simulink model "failure_detector"  (R2024b)
settings: Solver=VariableStepAuto  StartTime=0.0  StopTime=1  RelTol=1e-3
libraries: simulink x7, pil_lib x1
settings Model: Creator=bew  LastModifiedBy=bew

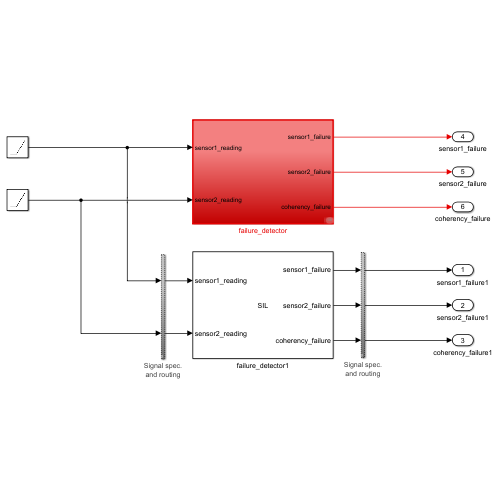
[thumbnail: Simulink's stored preview of the top-level diagram]
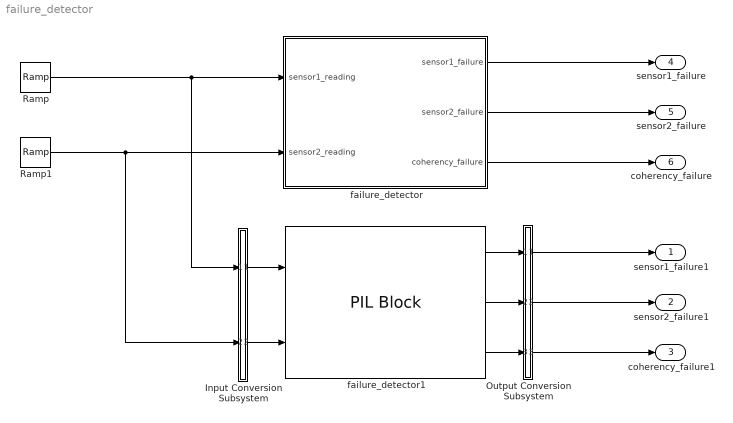
== system failure_detector ==
  Input Conversion Subsystem : Subsystem  Tag=__SLT_ICS__  Description=|
      | Signal spec.
      | and routing
      settings: AttributesFormatString=%<Description>
  Output Conversion Subsystem : Subsystem  Tag=__SLT_OCS__  Description=|
      | Signal spec.
      | and routing
      settings: AttributesFormatString=%<Description>
  Ramp : simulink/Sources/Ramp  slope=4  start=0  InitialOutput=0.5
  Ramp1 : simulink/Sources/Ramp  slope=-4  start=0  InitialOutput=4.5
  failure_detector : Subsystem  TreatAsAtomicUnit=on
  failure_detector1 : pil_lib/PIL Block  Tag=__SL_testing_harness_stub_  SimulationMode=SIL  IsTopModelPIL=off  CodeDir=D:\MBD_challenge\failure_detector_ert_rtw  AnchorDir=D:\MBD_challenge\xrel  ConfigName=Software-in-the-Loop (SIL)  XRelSourceFile=D:\MBD_challenge\failure_detector_ert_rtw\ert_main.c  XrelIsTopModelCode=on  XrelIsReusable=off  XrelDWorkNames={}  XrelDWorkTypes={}  XrelModelArgVals={}  XrelOrderedParamNames={}  XILSFunction=failure_detector_R2024b_sil  XRelNonFiniteStyle=NONFINITE_UNUSED
  sensor1_failure1 : Outport
  sensor2_failure1 : Outport  Port=2
  coherency_failure1 : Outport  Port=3
  sensor1_failure : Outport  Port=4
  sensor2_failure : Outport  Port=5
  coherency_failure : Outport  Port=6
  wires:
  Input Conversion Subsystem/1(Outport_1) -> failure_detector1/1
  Input Conversion Subsystem/2(Outport_2) -> failure_detector1/2
  failure_detector1/3 -> Output Conversion Subsystem/3(Inport_3)
  Output Conversion Subsystem/2(Outport_2) -> sensor2_failure1/1
  failure_detector1/2 -> Output Conversion Subsystem/2(Inport_2)
  Output Conversion Subsystem/1(Outport_1) -> sensor1_failure1/1
  failure_detector1/1 -> Output Conversion Subsystem/1(Inport_1)
  Output Conversion Subsystem/3(Outport_3) -> coherency_failure1/1
  failure_detector/1(sensor1_failure) -> sensor1_failure/1
  failure_detector/2(sensor2_failure) -> sensor2_failure/1
  failure_detector/3(coherency_failure) -> coherency_failure/1
  Ramp/1 -> Input Conversion Subsystem/1(Inport_1), failure_detector/1(sensor1_reading)
  Ramp1/1 -> Input Conversion Subsystem/2(Inport_2), failure_detector/2(sensor2_reading)

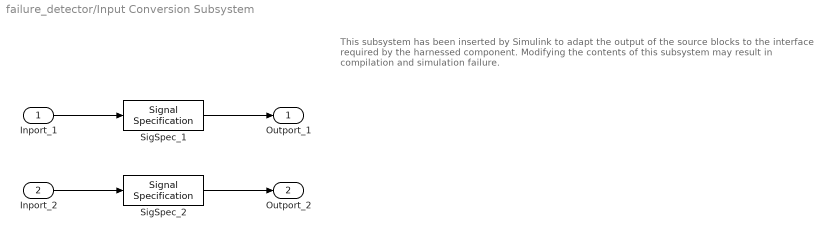
== system failure_detector/Input Conversion Subsystem ==
  note: This subsystem has been inserted by Simulink to adapt the output of the source blocks to the interface required by the harnessed component.
      |  Modifying the contents of this subsystem may result in compilation and simulation failure.
  Inport_1 : Inport
  Inport_2 : Inport  Port=2
  SigSpec_1 : SignalSpecification  OutDataTypeStr=double  Dimensions=[1]  SampleTime=0.2
  SigSpec_2 : SignalSpecification  OutDataTypeStr=double  Dimensions=[1]  SampleTime=0.2
  Outport_1 : Outport
  Outport_2 : Outport  Port=2
  wires:
  SigSpec_1/1 -> Outport_1/1
  Inport_1/1 -> SigSpec_1/1
  SigSpec_2/1 -> Outport_2/1
  Inport_2/1 -> SigSpec_2/1

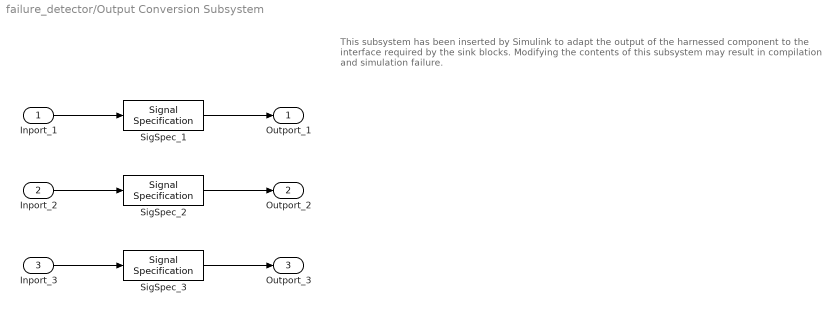
== system failure_detector/Output Conversion Subsystem ==
  note: This subsystem has been inserted by Simulink to adapt the output of the harnessed component to the interface required by the sink blocks.
      |  Modifying the contents of this subsystem may result in compilation and simulation failure.
  Inport_1 : Inport
  Inport_2 : Inport  Port=2
  Inport_3 : Inport  Port=3
  SigSpec_1 : SignalSpecification  OutDataTypeStr=boolean  Dimensions=[1]  SampleTime=0.2
  SigSpec_2 : SignalSpecification  OutDataTypeStr=boolean  Dimensions=[1]  SampleTime=0.2
  SigSpec_3 : SignalSpecification  OutDataTypeStr=boolean  Dimensions=[1]  SampleTime=0.2
  Outport_1 : Outport
  Outport_2 : Outport  Port=2
  Outport_3 : Outport  Port=3
  wires:
  Inport_1/1 -> SigSpec_1/1
  SigSpec_1/1 -> Outport_1/1
  Inport_2/1 -> SigSpec_2/1
  SigSpec_2/1 -> Outport_2/1
  Inport_3/1 -> SigSpec_3/1
  SigSpec_3/1 -> Outport_3/1

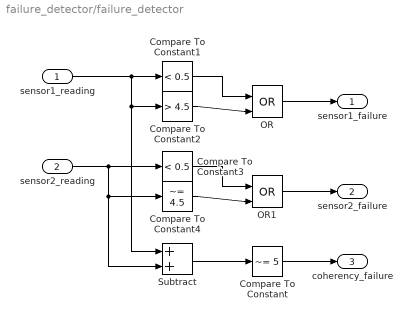
== system failure_detector/failure_detector ==
  sensor1_reading : Inport
  sensor2_reading : Inport  Port=2
  Compare To Constant : simulink/Logic and Bit Operations/Compare To Constant  relop=~=  const=5  OutDataTypeStr=boolean
  Compare To Constant1 : simulink/Logic and Bit Operations/Compare To Constant  relop=<  const=0.5  OutDataTypeStr=boolean
  Compare To Constant2 : simulink/Logic and Bit Operations/Compare To Constant  relop=>  const=4.5  OutDataTypeStr=boolean
  Compare To Constant3 : simulink/Logic and Bit Operations/Compare To Constant  relop=<  const=0.5  OutDataTypeStr=boolean
  Compare To Constant4 : simulink/Logic and Bit Operations/Compare To Constant  relop=~=  const=4.5  OutDataTypeStr=boolean
  OR : Logic  Operator=OR  IconShape=distinctive  AllPortsSameDT=off  OutDataTypeStr=boolean
  OR1 : Logic  Operator=OR  IconShape=distinctive  AllPortsSameDT=off  OutDataTypeStr=boolean
  Subtract : Sum
  sensor1_failure : Outport
  sensor2_failure : Outport  Port=2
  coherency_failure : Outport  Port=3
  wires:
  Compare To Constant1/1 -> OR/1
  Compare To Constant4/1 -> OR1/2
  Compare To Constant2/1 -> OR/2
  sensor2_reading/1 -> Subtract/2, Compare To Constant4/1, Compare To Constant3/1
  Compare To Constant3/1 -> OR1/1
  Subtract/1 -> Compare To Constant/1
  sensor1_reading/1 -> Subtract/1, Compare To Constant2/1, Compare To Constant1/1
  Compare To Constant/1 -> coherency_failure/1
  OR/1 -> sensor1_failure/1
  OR1/1 -> sensor2_failure/1
